simulink model "BMM_SingleElement"  (R2018a)
settings: Solver=VariableStepAuto  StartTime=0.0  StopTime=0.05  FixedStep=1/48000  RelTol=1e-3
model workspace (MAT data in the model file):
  C_1 = 1e-07
  C_6 = 5.7e-07
  L_0 = 0.033
  L_1 = 0.01
  L_6 = 0.01
  Ls_1 = 0.033
  R_1 = 150
  R_6 = 63
  U_inputGain = 1
libraries: powerlib x11, simulink x1
settings Model: Creator=rsalo  LastModifiedBy=Gerard

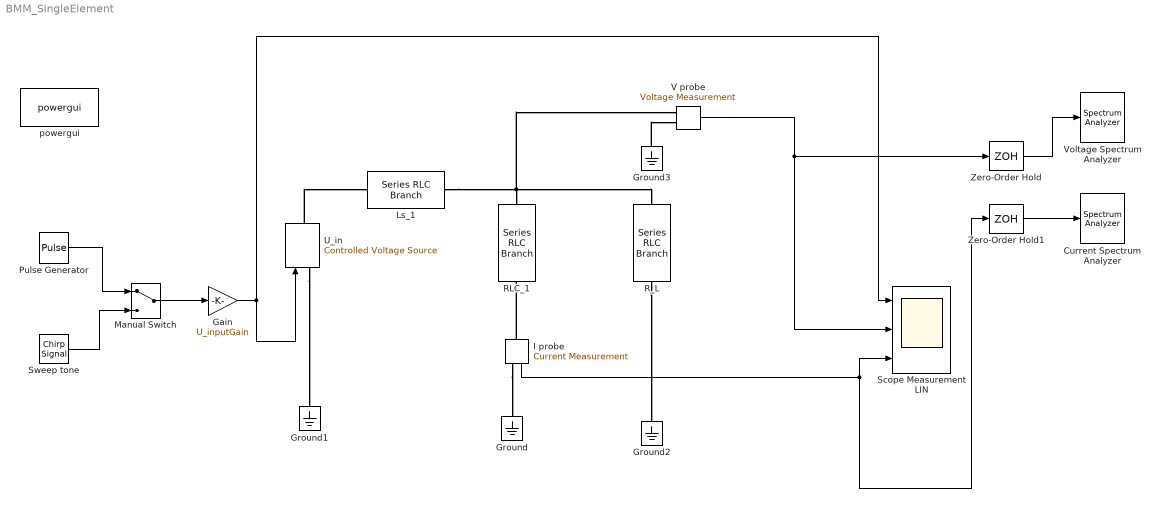
== system BMM_SingleElement ==
  Current Spectrum Analyzer : SpectrumAnalyzer
  Gain : Gain  Gain=U_inputGain
  Ground{,1..3} (4 alike) : powerlib/Elements/Ground  LConnTagsString=a
      settings: SourceProductName=Simscape Electrical
  I probe : powerlib/Measurements/Current Measurement  PhasorSimulation=off  OutputType=Complex  PSBequivalent=0
      settings: SourceProductName=Simscape Electrical
  Ls_1 : powerlib/Elements/Series RLC Branch  LConnTagsString=__new0  RConnTagsString=__new0  BranchType=L  Resistance=0  Inductance=Ls_1  SetiL0=off  InitialCurrent=0  Capacitance=0  Setx0=off  InitialVoltage=0  Measurements=None
      settings: SourceProductName=Simscape Electrical
  Manual Switch : ManualSwitch
  "Pulse Generator " : DiscretePulseGenerator  PulseType=Time based  Period=1  PulseWidth=0.001  SampleTime=1/48000
  RLC_1 : powerlib/Elements/Series RLC Branch  LConnTagsString=__new0  RConnTagsString=__new0  BranchType=RLC  Resistance=R_1  Inductance=L_1  SetiL0=off  InitialCurrent=0  Capacitance=C_1  Setx0=off  InitialVoltage=0  Measurements=None
      settings: SourceProductName=Simscape Electrical
  R_L : powerlib/Elements/Series RLC Branch  LConnTagsString=__new0  RConnTagsString=__new0  BranchType=R  Resistance=100  Inductance=1e-3  SetiL0=off  InitialCurrent=0  Capacitance=1e-6  Setx0=off  InitialVoltage=0  Measurements=None
      settings: SourceProductName=Simscape Electrical
  "Scope Measurement LIN " : Scope  NumInputPorts=3
  Sweep tone : simulink/Sources/Chirp Signal  f1=20  T=1  f2=10000
  U_in : powerlib/Electrical Sources/Controlled Voltage Source  Initialize=on  Source_Type=AC  Amplitude=0  Phase=0  Frequency=0  Measurements=None
      settings: SourceProductName=Simscape Electrical
  V probe : powerlib/Measurements/Voltage Measurement  PhasorSimulation=off  OutputType=Complex  PSBequivalent=0
      settings: SourceProductName=Simscape Electrical
  Voltage Spectrum Analyzer : SpectrumAnalyzer
  Zero-Order Hold : ZeroOrderHold  SampleTime=-1
  Zero-Order Hold1 : ZeroOrderHold  SampleTime=-1
  powergui : powerlib/powergui  Priority=1  SimulationMode=Discrete  SampleTime=50e-6  frequency=60  Iterations=50  frequencyindice=0  Pbase=100e6  ErrMax=1e-4  UnitsV=kV  UnitsW=MW  buscounter=0  FunctionMessages=off  echomessages=off  EnableUseOfTLC=off  CurrentSourceSwitches=off  DisableSnubberDevices=off  DisableRonSwitches=off  DisableVfSwitches=off  DisplayEquations=off  SolverType=Tustin/Backward Euler (TBE)  Interpol=off  ExternalGateDelay=off  methode=off  Ts=100  x0status=blocks  SPID=off  SwTol=0  HookPort=off  RestoreLinks=warning  ResistiveCurrentMeasurement=off  Frange=[0:2:500]  Ylog=off  Xlog=on  ShowGrid=off  save=off  variable=ZData  structure=0  ZoomFFT=off  StartTime=0.0  cycles=1  DisplayStyle=1  fundamental=60  FreqAxis=off  MaxFrequency=1000  frequencyindicesteady=1  RmsSteady=1  display=off
  wires:
  Manual Switch/1 -> Gain/1
  Gain/1 -> "Scope Measurement LIN "/1, U_in/1
  V probe/1 -> "Scope Measurement LIN "/2, Zero-Order Hold/1
  I probe/1 -> Zero-Order Hold1/1, "Scope Measurement LIN "/3
  Sweep tone/1 -> Manual Switch/2
  "Pulse Generator "/1 -> Manual Switch/1
  Zero-Order Hold/1 -> Voltage Spectrum Analyzer/1
  Zero-Order Hold1/1 -> Current Spectrum Analyzer/1
  connections:
  U_in/RConn1 -- Ls_1/LConn1
  Ls_1/RConn1 -- R_L/RConn1 -- V probe/LConn1 -- RLC_1/RConn1
  I probe/RConn1 -- Ground/LConn1
  I probe/LConn1 -- RLC_1/LConn1
  U_in/LConn1 -- Ground1/LConn1
  R_L/LConn1 -- Ground2/LConn1
  Ground3/LConn1 -- V probe/LConn2
